simulink model "lqr1"  (R2013a)
settings: Solver=ode45  StartTime=0.0  StopTime=10  RelTol=1e-3
InitFcn:
  | A=A
  | B=B
  | C=C
settings Model: Creator=user  LastModifiedBy=user

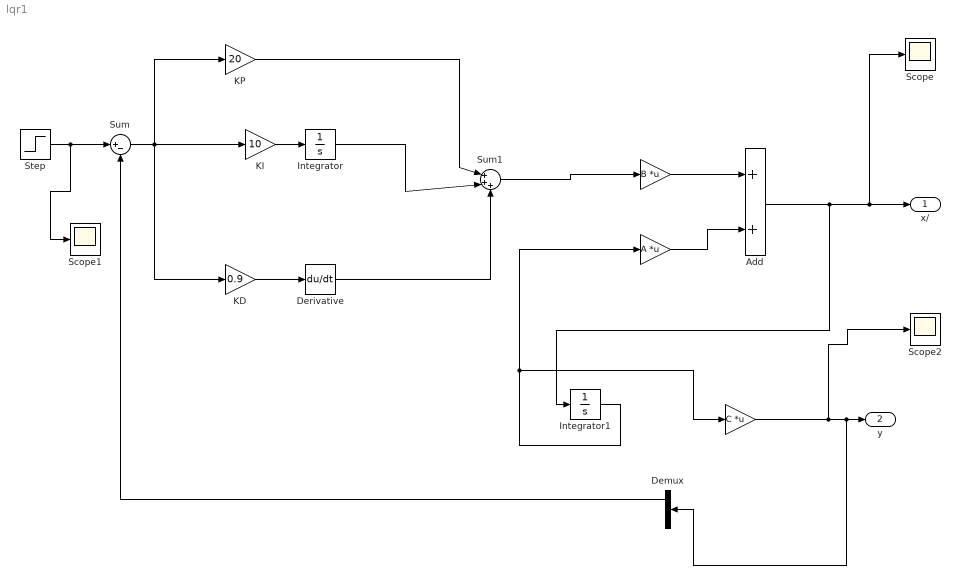
== system lqr1 ==
  " " : Gain  Gain=B  Multiplication=Matrix(K*u) (u vector)
  " " : Gain  Gain=A  Multiplication=Matrix(K*u) (u vector)
  " " : Gain  Gain=C  Multiplication=Matrix(K*u) (u vector)
  Add : Sum
  Demux : Demux  Outputs=2
  Derivative : Derivative
  Integrator : Integrator
  Integrator1 : Integrator
  KD : Gain  Gain=0.9
  KI : Gain  Gain=10
  KP : Gain  Gain=20
  Scope : Scope
  Scope1 : Scope
  Scope2 : Scope
      settings: SaveName=ScopeData2
  Step : Step  After=90  SampleTime=1
  Sum : Sum  Inputs=|+-
  Sum1 : Sum  Inputs=|+++
  "x/ " : Outport
  y : Outport  Port=2
  wires:
  KP/1 -> Sum1/1
  Integrator/1 -> Sum1/2
  Derivative/1 -> Sum1/3
  Sum/1 -> KD/1, KI/1, KP/1
  KI/1 -> Integrator/1
  KD/1 -> Derivative/1
  " "/1 -> Add/1
  " "/1 -> Add/2
  " "/1 -> Scope2/1, Demux/1, y/1
  Sum1/1 -> " "/1
  Add/1 -> Integrator1/1, Scope/1, "x/ "/1
  Integrator1/1 -> " "/1, " "/1
  Step/1 -> Scope1/1, Sum/1
  Demux/1 -> Sum/2
